simulink model "sampleModel1654"  (R2023a)
settings: Solver=VariableStepAuto  StartTime=0.0  StopTime=10.0  RelTol=1e-3
libraries: hdlsllib x7, simulink x4
settings Model: Creator=user1  LastModifiedBy=user1

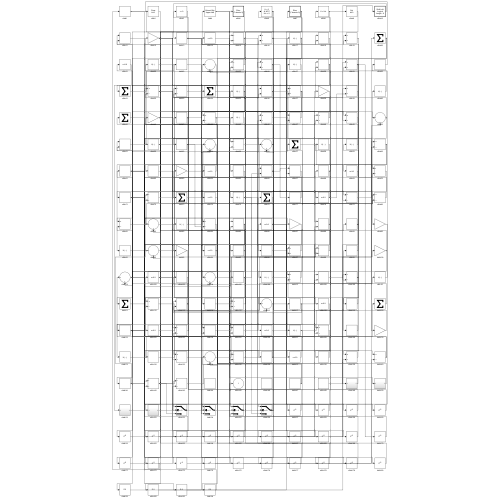
[thumbnail: Simulink's stored preview of the top-level diagram]
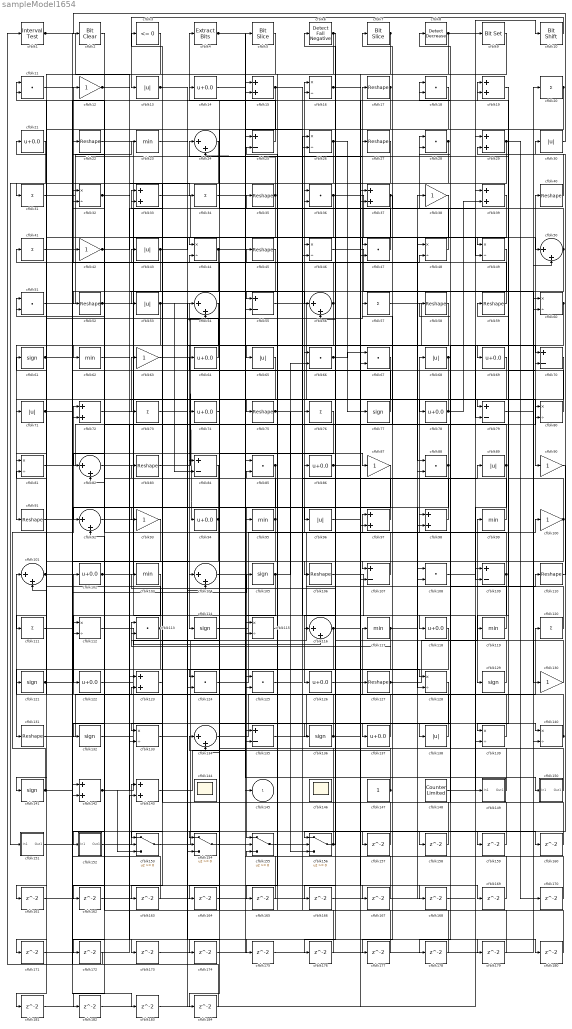
== system sampleModel1654 ==
  cfblk1 : hdlsllib/Logic and Bit Operations/Interval Test  IntervalClosedRight=on  uplimit=0.5  IntervalClosedLeft=on  lowlimit=-0.5  OutDataTypeStr=boolean
  cfblk10 : hdlsllib/Logic and Bit Operations/Bit Shift  mode=Shift Left Logical  N=0
  cfblk{12,38,42,63,87,90,93,100,130} (9 alike) : Gain
  cfblk{24,50,54,56,82,92,101,104,116,134} (10 alike) : Sum  Inputs=|++
  cfblk{14,21,64,69,74,78,86,94,102,118,122,126,137} (13 alike) : Bias  Bias=0.0  SaturateOnIntegerOverflow=off
  cfblk{23,62,95,99,103,117,119} (7 alike) : MinMax
  cfblk{61,77,105,114,121,129,132,136,141} (9 alike) : Signum
  cfblk{17,22,27,35,40,45,52,58..59,75,83,91,106,110,127,131} (16 alike) : Reshape
  cfblk{25,55,70,79,84,107,109,135} (8 alike) : Sum  Inputs=+-
  cfblk{11,18,28,36,47,51,66..67,85,88,108,113,124..125} (14 alike) : DotProduct  OutDataTypeStr=Inherit: Inherit via internal rule
  cfblk{20,31,34,41,57,73,76,111,120} (9 alike) : Sum  Inputs=+
  cfblk{16,26,32,44,46,48..49,60,80..81,112,115,128,133,139..140} (16 alike) : Product  Inputs=*/  RndMeth=Zero  SaturateOnIntegerOverflow=on
  cfblk{15,19,29,33,37,39,72,97..98,123,142..143} (12 alike) : Sum
  cfblk{13,30,43,53,65,68,71,89,96,138} (10 alike) : Abs  SaturateOnIntegerOverflow=off
  cfblk144 : Scope
      settings: Floating=on
  cfblk146 : Scope
      settings: Floating=on
  cfblk147 : Constant  SampleTime=-1
  cfblk148 : hdlsllib/Sources/Counter Limited  uplimit=7  tsamp=-1
  cfblk149 : Subsystem
      settings: LibrarySourceBlock=|
      | hdlsllib/Ports &
      | Subsystems/Subsystem
  cfblk150 : Subsystem
      settings: LibrarySourceBlock=|
      | hdlsllib/Ports &
      | Subsystems/Subsystem
  cfblk151 : Subsystem
      settings: LibrarySourceBlock=|
      | hdlsllib/Ports &
      | Subsystems/Subsystem
  cfblk152 : Subsystem
      settings: LibrarySourceBlock=|
      | hdlsllib/Ports &
      | Subsystems/Subsystem
  cfblk{153..156} (4 alike) : Switch  SaturateOnIntegerOverflow=off  InputSameDT=off
  cfblk{157..184} (28 alike) : Delay  SampleTime=1
  cfblk2 : simulink/Logic and Bit Operations/Bit Clear  iBit=0
      settings: LibrarySourceBlock=|
      | hdlsllib/Logic and Bit
      | Operations/Bit Clear
  cfblk3 : hdlsllib/Logic and Bit Operations/Compare To Zero  relop=<=  OutDataTypeStr=boolean
  cfblk4 : simulink/Logic and Bit Operations/Extract Bits  bitsToExtract=Upper half  numBits=8  bitIdxRange=[0 7]  outScalingMode=Preserve fixed-point scaling
      settings: LibrarySourceBlock=|
      | hdlsllib/Logic and Bit
      | Operations/Extract Bits
  cfblk5 : hdlsllib/Logic and Bit Operations/Bit Slice  lidx=7  ridx=0
  cfblk6 : hdlsllib/Logic and Bit Operations/Detect Fall Negative  vinit=0  OutDataTypeStr=boolean
  cfblk7 : hdlsllib/Logic and Bit Operations/Bit Slice  lidx=7  ridx=0
  cfblk8 : simulink/Logic and Bit Operations/Detect Decrease  vinit=0.0  OutDataTypeStr=boolean
      settings: LibrarySourceBlock=|
      | hdlsllib/Logic and Bit
      | Operations/Detect
      | Decrease
  cfblk9 : simulink/Logic and Bit Operations/Bit Set  iBit=0
      settings: LibrarySourceBlock=|
      | hdlsllib/Logic and Bit
      | Operations/Bit Set
  cfblk145 : Outport  VectorParamsAs1DForOutWhenUnconnected=off
  wires:
  cfblk58/1 -> cfblk114/1
  cfblk59/1 -> cfblk12/1
  cfblk97/1 -> cfblk22/1
  cfblk85/1 -> cfblk155/1, cfblk154/2
  cfblk25/1 -> cfblk4/1
  cfblk118/1 -> cfblk131/1
  cfblk150/1(Out1) -> cfblk113/1
  cfblk139/1 -> cfblk102/1
  cfblk120/1 -> cfblk24/1
  cfblk107/1 -> cfblk16/1
  cfblk54/1 -> cfblk91/1
  cfblk78/1 -> cfblk75/1, cfblk39/2
  cfblk10/1 -> cfblk13/1
  cfblk142/1 -> cfblk25/1, cfblk80/2, cfblk153/3
  cfblk141/1 -> cfblk72/1, cfblk66/1, cfblk175/1
  cfblk53/1 -> cfblk94/1, cfblk84/2, cfblk62/1
  cfblk66/1 -> cfblk67/1, cfblk166/1
  cfblk63/1 -> cfblk46/1
  cfblk100/1 -> cfblk19/1, cfblk153/1
  cfblk44/1 -> cfblk152/1(In1), cfblk36/2
  cfblk22/1 -> cfblk126/1
  cfblk103/1 -> cfblk122/1
  cfblk98/1 -> cfblk3/1
  cfblk83/1 -> cfblk17/1
  cfblk130/1 -> cfblk76/1
  cfblk23/1 -> cfblk67/2
  cfblk31/1 -> cfblk27/1
  cfblk50/1 -> cfblk28/1, cfblk134/2
  cfblk153/1 -> cfblk97/1
  cfblk123/1 -> cfblk33/1
  cfblk90/1 -> cfblk156/1
  cfblk137/1 -> cfblk117/1
  cfblk102/1 -> cfblk9/1, cfblk169/1
  cfblk52/1 -> cfblk79/1, cfblk182/1
  cfblk49/1 -> cfblk72/2
  cfblk115/1 -> cfblk35/1
  cfblk55/1 -> cfblk90/1
  cfblk81/1 -> cfblk40/1
  cfblk72/1 -> cfblk63/1
  cfblk36/1 -> cfblk50/1, cfblk133/1
  cfblk92/1 -> cfblk127/1
  cfblk138/1 -> cfblk101/1
  cfblk135/1 -> cfblk120/1
  cfblk119/1 -> cfblk8/1
  cfblk37/1 -> cfblk95/1, cfblk107/1, cfblk96/1
  cfblk129/1 -> cfblk103/1
  cfblk56/1 -> cfblk43/1, cfblk133/2
  cfblk21/1 -> cfblk151/1(In1)
  cfblk84/1 -> cfblk112/1
  cfblk124/1 -> cfblk68/1
  cfblk114/1 -> cfblk50/2
  cfblk24/1 -> cfblk121/1
  cfblk26/1 -> cfblk53/1, cfblk77/1
  cfblk69/1 -> cfblk71/1
  cfblk87/1 -> cfblk125/1
  cfblk116/1 -> cfblk98/1, cfblk135/2
  cfblk65/1 -> cfblk111/1
  cfblk82/1 -> cfblk48/1
  cfblk57/1 -> cfblk79/2
  cfblk39/1 -> cfblk81/1
  cfblk140/1 -> cfblk58/1, cfblk51/2
  cfblk96/1 -> cfblk19/2
  cfblk155/1 -> cfblk89/1
  cfblk20/1 -> cfblk106/1, cfblk37/2
  cfblk104/1 -> cfblk5/1
  cfblk86/1 -> cfblk159/1, cfblk160/1
  cfblk71/1 -> cfblk140/1, cfblk157/1, cfblk158/1
  cfblk75/1 -> cfblk118/1, cfblk156/3
  cfblk15/1 -> cfblk44/1, cfblk97/2
  cfblk134/1 -> cfblk38/1
  cfblk108/1 -> cfblk39/1
  cfblk61/1 -> cfblk112/2, cfblk87/1, cfblk173/1
  cfblk122/1 -> cfblk20/1
  cfblk131/1 -> cfblk15/2
  cfblk101/1 -> cfblk104/1, cfblk70/2
  cfblk40/1 -> cfblk29/2
  cfblk1/1 -> cfblk123/1, cfblk93/1
  cfblk149/1(Out1) -> cfblk41/1
  cfblk89/1 -> cfblk57/1, cfblk109/2
  cfblk109/1 -> cfblk129/1, cfblk11/1
  cfblk11/1 -> cfblk98/2
  cfblk111/1 -> cfblk48/2
  cfblk2/1 -> cfblk82/1
  cfblk16/1 -> cfblk116/1, cfblk168/1
  cfblk17/1 -> cfblk115/2, cfblk47/2
  cfblk47/1 -> cfblk14/1
  cfblk51/1 -> cfblk23/1
  cfblk38/1 -> cfblk82/2
  cfblk110/1 -> cfblk30/1
  cfblk156/1 -> cfblk86/1, cfblk83/1
  cfblk105/1 -> cfblk125/2, cfblk66/2
  cfblk93/1 -> cfblk101/2
  cfblk143/1 -> cfblk85/1
  cfblk74/1 -> cfblk124/1
  cfblk147/1 -> cfblk42/1, cfblk134/1
  cfblk42/1 -> cfblk56/1, cfblk36/1
  cfblk106/1 -> cfblk149/1(In1)
  cfblk132/1 -> cfblk104/2
  cfblk48/1 -> cfblk7/1
  cfblk60/1 -> cfblk69/1, cfblk138/1
  cfblk127/1 -> cfblk99/1, cfblk177/1
  cfblk154/1 -> cfblk145/1
  cfblk125/1 -> cfblk46/2
  cfblk19/1 -> cfblk119/1
  cfblk6/1 -> cfblk55/1, cfblk176/1
  cfblk4/1 -> cfblk26/2, cfblk150/1(In1)
  cfblk68/1 -> cfblk137/1, cfblk18/2
  cfblk64/1 -> cfblk21/1
  cfblk7/1 -> cfblk132/1, cfblk107/2
  cfblk30/1 -> cfblk2/1
  cfblk41/1 -> cfblk84/1
  cfblk117/1 -> cfblk108/1, cfblk113/2, cfblk174/1
  cfblk112/1 -> cfblk116/2
  cfblk95/1 -> cfblk51/1, cfblk181/1
  cfblk126/1 -> cfblk80/1
  cfblk79/1 -> cfblk60/1
  cfblk46/1 -> cfblk130/1
  cfblk12/1 -> cfblk74/1, cfblk34/1, cfblk136/1
  cfblk18/1 -> cfblk141/1
  cfblk151/1(Out1) -> cfblk18/1
  cfblk34/1 -> cfblk70/1
  cfblk77/1 -> cfblk64/1
  cfblk113/1 -> cfblk61/1, cfblk172/1
  cfblk5/1 -> cfblk31/1
  cfblk152/1(Out1) -> cfblk143/1
  cfblk136/1 -> cfblk110/1, cfblk81/2, cfblk11/2
  cfblk14/1 -> cfblk49/1
  cfblk43/1 -> cfblk142/2, cfblk47/1
  cfblk28/1 -> cfblk56/2, cfblk154/3
  cfblk32/1 -> cfblk73/1, cfblk49/2
  cfblk13/1 -> cfblk16/2, cfblk54/2, cfblk128/1
  cfblk94/1 -> cfblk92/1, cfblk153/2
  cfblk121/1 -> cfblk45/1, cfblk105/1, cfblk167/1
  cfblk73/1 -> cfblk78/1
  cfblk99/1 -> cfblk6/1
  cfblk29/1 -> cfblk139/1, cfblk170/1, cfblk171/1
  cfblk35/1 -> cfblk154/1, cfblk124/2, cfblk24/2
  cfblk8/1 -> cfblk52/1, cfblk10/1
  cfblk80/1 -> cfblk59/1
  cfblk88/1 -> cfblk32/2, cfblk128/2
  cfblk33/1 -> cfblk88/1
  cfblk9/1 -> cfblk65/1
  cfblk148/1 -> cfblk100/1
  cfblk157/1 -> cfblk15/1
  cfblk158/1 -> cfblk123/2
  cfblk159/1 -> cfblk33/2
  cfblk160/1 -> cfblk28/2
  cfblk27/1 -> cfblk161/1
  cfblk161/1 -> cfblk108/2
  cfblk3/1 -> cfblk162/1
  cfblk162/1 -> cfblk29/1
  cfblk45/1 -> cfblk163/1
  cfblk163/1 -> cfblk142/1
  cfblk76/1 -> cfblk164/1
  cfblk164/1 -> cfblk135/1
  cfblk67/1 -> cfblk165/1
  cfblk165/1 -> cfblk115/1
  cfblk166/1 -> cfblk88/2
  cfblk167/1 -> cfblk156/2
  cfblk168/1 -> cfblk139/2
  cfblk169/1 -> cfblk155/3
  cfblk170/1 -> cfblk85/2
  cfblk171/1 -> cfblk143/2
  cfblk172/1 -> cfblk1/1
  cfblk173/1 -> cfblk55/2
  cfblk174/1 -> cfblk60/2
  cfblk175/1 -> cfblk140/2
  cfblk176/1 -> cfblk92/2
  cfblk177/1 -> cfblk25/2
  cfblk70/1 -> cfblk178/1
  cfblk178/1 -> cfblk44/2
  cfblk62/1 -> cfblk179/1
  cfblk179/1 -> cfblk26/1
  cfblk133/1 -> cfblk180/1
  cfblk180/1 -> cfblk155/2
  cfblk181/1 -> cfblk37/1
  cfblk182/1 -> cfblk109/1
  cfblk91/1 -> cfblk183/1
  cfblk183/1 -> cfblk54/1
  cfblk128/1 -> cfblk184/1
  cfblk184/1 -> cfblk32/1

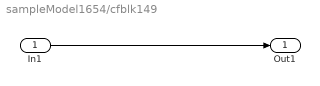
== system sampleModel1654/cfblk149 ==
  In1 : Inport
  Out1 : Outport
  wires:
  In1/1 -> Out1/1

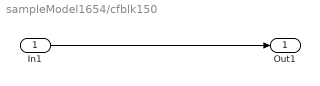
== system sampleModel1654/cfblk150 ==
  In1 : Inport
  Out1 : Outport
  wires:
  In1/1 -> Out1/1

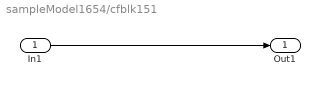
== system sampleModel1654/cfblk151 ==
  In1 : Inport
  Out1 : Outport
  wires:
  In1/1 -> Out1/1

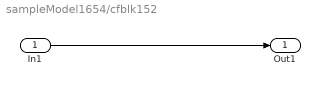
== system sampleModel1654/cfblk152 ==
  In1 : Inport
  Out1 : Outport
  wires:
  In1/1 -> Out1/1
